simulink model "Main_plasticbike"  (R2022b)
settings: Solver=ode23  StartTime=0.0  StopTime=sim_time-0.02
undefined symbols (not defined in the file): bike_model, bike_params, D_balancing_inner, D_balancing_outer, e1_max, g, I_balancing_inner, I_balancing_outer, initial_state, k1, k2, linearized_sys, P_balancing_inner, P_balancing_outer, pert_deltadot_state, pert_deltadot_state_fun, pert_phidot_state, pert_phidot_state_fun, Psiref, Th, Ts, v, Xref, Yref
libraries: slpidlib x2, cstblocks x1
settings Model: Creator=Hadi Hajieghrary  LastModifiedBy=levi1
settings SolverCC: MaxConsecutiveMinStep=10  ZeroCrossAlgorithm=Adaptive  AlgebraicLoopSolver=TrustRegion  AutoInsertRateTranBlk=on
settings DebuggingCC: AlgebraicLoopMsg=none  UnconnectedInputMsg=warning  UnconnectedOutputMsg=warning  UnconnectedLineMsg=warning
settings ModelReferenceCC: EnableRefExpFcnMdlSchedulingChecks=on
settings RTWCC: DLArmComputeVersion=19.05

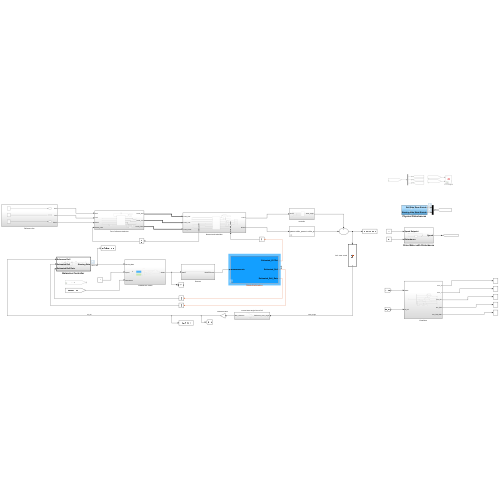
[thumbnail: Simulink's stored preview of the top-level diagram]
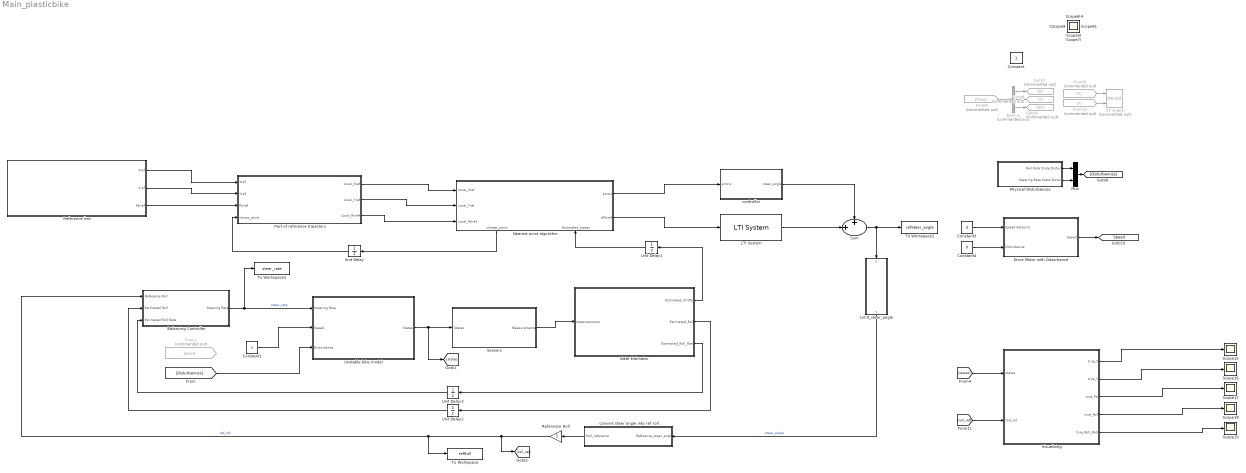
== system Main_plasticbike ==
  "Balancing Controller " : Subsystem  TreatAsAtomicUnit=on  SystemSampleTime=Ts
      settings: MinAlgLoopOccurrences=on
  Constant1 : Constant  Value=v
  Constant3 : Constant  Value=3
  Constant4 : Constant  Value=0
  Demux : Demux  Commented=on  Outputs=3
  Drive Motor with Disturbance : Subsystem
  From1 : From  Commented=on  GotoTag=Speed  TagVisibility=global
  From10 : From  Commented=on  GotoTag=Y
  From8 : From  Commented=on  GotoTag=Pose
  From9 : From  Commented=on  GotoTag=X
  Goto7 : Goto  Commented=on  GotoTag=X
  Goto8 : Goto  Commented=on  GotoTag=Y
  Goto9 : Goto  Commented=on  GotoTag=psi
  LTI System : cstblocks/LTI System  sys=tf(1,[bike_params.a/bike_params.b v/bike_params.b])  IC=[]
  Limit_steer_angle : MATLAB Function  TreatAsAtomicUnit=on
  Mux : Mux  Inputs=2
  Nearest point algorithm : Subsystem
      settings: PortSchema="{\"entries\":[{\"content\":{\"sides\":[{\"content\":{\"connectorIds\":[\"In1\",\"In2\",\"In3\"]},\"type\":\"ConnectorPlacement.EquallySpacedRectSide\",\"uuid\":\"cc846df4-97c1-4e38-a551-63d96742d514\"},{\"content\":{\"connectorIds\":[\"Out1\",\"Out2\"],\"side\":\"RIGHT\"},\"type\":\"ConnectorPlacement.EquallySpacedRectSide\",\"uuid\":\"926eeee4-c51a-40d9-a9a1-df7a0c76cd55\"},{\"content\":{\"connectorIds\":[],\"side\":\"TOP\"},\"type\":\"ConnectorPlacement.EquallySpacedRectSide\",\"uuid\":\"e902e63c-5309-44b2-99e1-76b44c06d1f2\"},{\"content\":{\"connectorIds\":[\"Out3\",\"In4\"],\"side\":\"BOTTOM\"},\"type\":\"ConnectorPlacement.EquallySpacedRectSide\",\"uuid\":\"f92d60b4-b11f-4907-83c4-1907c5b6c496\"}]},\"type\":\"ConnectorPlacement.EquallySpacedConnector\",\"uuid\":\"17b67b4e-0a47-44a6-bf11-0cf8a9b1982c\"}],\"packageUris\":[\"http://schema.mathworks.com/mf0/Connector/R2020b\"],\"version\":\"1.0\"}"
  Part of reference trajectory : Subsystem
  Physical Disturbances : Subsystem
  Reference Roll : Gain
  Reference line : Subsystem
  Scope{,1..19} (20 alike) : Scope
  Sensors : Subsystem
  State Estimator : Subsystem  mask{Parameters=bike_params, Initial_State=initial_state}
      mask prompts: Initial_State "Initial State"
  Sum : Sum  Inputs=++|
  To Workspace : ToWorkspace  VariableName=refRoll  SaveFormat=Timeseries  SampleTime=-1
  To Workspace1 : ToWorkspace  VariableName=refSteer_angle  SaveFormat=Timeseries  SampleTime=-1
  To Workspace2 : ToWorkspace  VariableName=steer_rate  SaveFormat=Timeseries  SampleTime=-1
  Unit Delay : UnitDelay  InitialCondition=1  SampleTime=Ts  HasFrameUpgradeWarning=on
  Unit Delay1 : UnitDelay  InitialCondition=[initial_state.x,initial_state.y,initial_state.heading]  SampleTime=Ts  HasFrameUpgradeWarning=on
  Unit Delay2 : UnitDelay  InitialCondition=initial_state.roll  SampleTime=Ts  HasFrameUpgradeWarning=on
  Unit Delay3 : UnitDelay  InitialCondition=initial_state.roll_rate  SampleTime=Ts  HasFrameUpgradeWarning=on
  Unstable bike model : Subsystem
  Visualizing : Subsystem
  XY Graph : Record  Commented=on  FileSettingsInternal="{\"entries\":[{\"content\":{\"excelSettings\":{\"content\":{},\"type\":\"Streamout.ExcelSettings\"}},\"type\":\"Streamout.FileSettingStorage\",\"uuid\":\"b0b94e94-796c-45bd-bc66-13715b3cee68\"}],\"packageUris\":[\"http://schema.mathworks.com/mf0/streamout_blocks/R2020a\"],\"version\":\"1.0\"}"  Layout=[1 1]  SignalsInternal="{\"entries\":[{\"content\":{\"signals\":[]},\"type\":\"RecordBlkView.InputSignals\",\"uuid\":\"7ae09d58-3f85-47c3-a863-15e07ca78b5f\"}],\"packageUris\":[\"http://schema.mathworks.com/mf0/streamout_blocks/R2020a\"],\"version\":\"1.0\"}"  VisualizationBindings="{\"xyplotplugin\":{\"info\":[{\"series\":[],\"subplotID\":1}]}}"  CompatibilityTag=XY
  controller : Subsystem
  convert steer angle into ref roll : Subsystem
  Constant : Constant  IOType=siggen
  tag scope: Speed=global
  wires:
  From8/1 -> Demux/1
  Demux/1 -> Goto7/1
  Demux/2 -> Goto8/1
  Demux/3 -> Goto9/1
  From10/1 -> XY Graph/2
  From9/1 -> XY Graph/1
  Physical Disturbances/1(Roll Rate State Disturb) -> Mux/1
  Physical Disturbances/2(Steering Rate State Disturb) -> Mux/2
  Mux/1 -> [Disturbances]
  Drive Motor with Disturbance/1(Speed) -> [Speed]
  Constant3/1 -> Drive Motor with Disturbance/1(Speed Setpoint)
  Constant4/1 -> Drive Motor with Disturbance/2(Disturbance)
  "Balancing Controller "/1(Steering Rate) -> Unstable bike model/1(Steering Rate), To Workspace2/1  "steer_rate"
  Reference line/1(Xref) -> Part of reference trajectory/1(Xref)
  Part of reference trajectory/1(Local_Xref) -> Nearest point algorithm/1(Local_Xref)
  Nearest point algorithm/3(closest_point) -> Unit Delay/1
  Nearest point algorithm/1(errors) -> controller/1(errors)
  Unit Delay/1 -> Part of reference trajectory/4(closes_point)
  controller/1(steer_angle) -> Sum/1
  LTI System/1 -> Sum/2
  Nearest point algorithm/2(dPsiref) -> LTI System/1
  Sum/1 -> Limit_steer_angle/1(u), To Workspace1/1
  Limit_steer_angle/1(y) -> convert steer angle into ref roll/1(Reference_steer_angle)  "steer_angle"
  convert steer angle into ref roll/1(Roll_reference) -> Reference Roll/1
  Reference Roll/1 -> [roll_ref], To Workspace/1, "Balancing Controller "/1(Reference Roll)  "ref_roll"
  [Disturbances] -> Unstable bike model/3(Disturbance)
  State Estimator/1(Estimated_X/Y/Psi) -> Unit Delay1/1
  State Estimator/2(Estimated_Roll) -> Unit Delay2/1
  State Estimator/3(Estimated_Roll_Rate) -> Unit Delay3/1
  Sensors/1(Measurements) -> State Estimator/1(measurements)
  Part of reference trajectory/2(Local_Yref) -> Nearest point algorithm/2(Local_Yref)
  Part of reference trajectory/3(Local_Psiref) -> Nearest point algorithm/3(Local_Psiref)
  Reference line/3(Psiref) -> Part of reference trajectory/3(Psiref)
  [states] -> Visualizing/1(states)
  Visualizing/1(true_X) -> Scope15/1
  Visualizing/2(true_Y) -> Scope16/1
  Visualizing/3(true_Psi) -> Scope17/1
  Visualizing/4(true_Roll) -> Scope18/1
  Visualizing/5(true_Roll_Rate) -> Scope19/1
  Unit Delay1/1 -> Nearest point algorithm/4(Estimated_states)
  Unit Delay2/1 -> "Balancing Controller "/2(Estimated Roll)
  Unit Delay3/1 -> "Balancing Controller "/3(Estimated Roll Rate)
  Reference line/2(Yref) -> Part of reference trajectory/2(Yref)
  [roll_ref] -> Visualizing/2(roll_ref)
  Unstable bike model/1(States) -> [states], Sensors/1(States)
  Constant1/1 -> Unstable bike model/2(Speed)

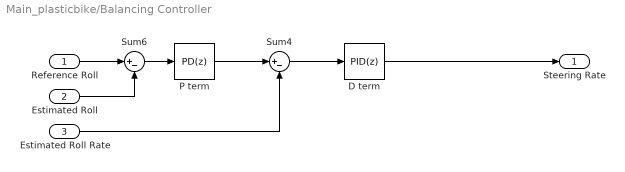
== system Main_plasticbike/Balancing Controller  ==
  Reference Roll : Inport
  Estimated Roll : Inport  Port=2
  Estimated Roll Rate : Inport  Port=3
  D term : slpidlib/PID Controller  Controller=PID  Form=Parallel  TimeDomain=Discrete-time  UseExternalTs=off  SampleTime=Ts  IntegratorMethod=Forward Euler  FilterMethod=Forward Euler  ControllerParametersSource=internal  P=P_balancing_inner  I=I_balancing_inner  UseKiTs=off  D=D_balancing_inner  N=100  UseFilter=off  TunerSelectOption=Transfer Function Based (PID Tuner App)  InitialConditionSource=internal  InitialConditionForIntegrator=0  InitialConditionForFilter=0  DifferentiatorICPrevScaledInput=0  ExternalReset=none  TrackingMode=off  Kt=1  LimitOutput=off  SatLimitsSource=internal  UpperSaturationLimit=inf  LowerSaturationLimit=-inf  LinearizeAsGain=on  AntiWindupMode=none  Kb=1  LimitIntegrator=off  UpperIntegratorSaturationLimit=inf  LowerIntegratorSaturationLimit=-inf  POutMin=[]  POutMax=[]  IOutMin=[]  IOutMax=[]  DOutMin=[]  DOutMax=[]  NOutMin=[]  NOutMax=[]  SumOutMin=[]  SumOutMax=[]  SaturationOutMin=[]  SaturationOutMax=[]  PParamMin=[]  PParamMax=[]  IParamMin=[]  IParamMax=[]  DParamMin=[]  DParamMax=[]  NParamMin=[]  NParamMax=[]  KbParamMin=[]  KbParamMax=[]  KtParamMin=[]  KtParamMax=[]  KbOutMin=[]  KbOutMax=[]  KtOutMin=[]  KtOutMax=[]  IntegratorOutMin=[]  IntegratorOutMax=[]  FilterOutMin=[]  FilterOutMax=[]  SumI1OutMin=[]  SumI1OutMax=[]  SumI2OutMin=[]  SumI2OutMax=[]  SumI3OutMin=[]  SumI3OutMax=[]  SumI4OutMin=[]  SumI4OutMax=[]  SumDOutMin=[]  SumDOutMax=[]  DifferentiatorOutMin=[]  DifferentiatorOutMax=[]  FilterDiffOutCoefMin=[]  FilterDiffOutCoefMax=[]  ReciprocalOutMin=[]  ReciprocalOutMax=[]  SumDenOutMin=[]  SumDenOutMax=[]  SumNumOutMin=[]  SumNumOutMax=[]  DivideOutMin=[]  DivideOutMax=[]  UdiffTsProdOutMin=[]  UdiffTsProdOutMax=[]  NTsProdOutMin=[]  NTsProdOutMax=[]  UintegralTsProdOutMin=[]  UintegralTsProdOutMax=[]  UngainTsProdOutMin=[]  UngainTsProdOutMax=[]  IntegratorContinuousStateAttributes=''  IntegratorStateMustResolveToSignalObject=off  IntegratorRTWStateStorageClass=Auto  FilterContinuousStateAttributes=''  FilterStateMustResolveToSignalObject=off  FilterRTWStateStorageClass=Auto  ParallelPVariant=InternalParameters  IdealPVariant=Disabled  IVariant=InternalParameters  DVariant=InternalParameters  IntegratorVariant=Discrete  SatVariant=Disabled  AWVariant=Passthrough  PCopyVariant=Disabled  TRVariant=Disabled  FdbkBlocksVariant=Forward  IdealPFdbkVariant=Disabled  SatFdbkVariant=Disabled  DerivativeFilterVariant=Differentiator  NVariant=Passthrough  NCopyVariant=Disabled_SignalSpec  FilterICVariant=InternalICsDifferentiator  IntegratorICVariant=InternalICs  ExternalResetVariant=Disabled  TRSumVariant=Passthrough  SumFdbkVariant=Disabled  SumVariant=Sum_PID  TsampFilterVariant=InternalTs  TsampNgainVariant=Passthrough  TsampIntegralVariant=Passthrough  ExternalSaturationOutDataTypeStr=Inherit: Same as second input
  P term : slpidlib/PID Controller  Controller=PD  Form=Parallel  TimeDomain=Discrete-time  UseExternalTs=off  SampleTime=Ts  IntegratorMethod=Forward Euler  FilterMethod=Forward Euler  ControllerParametersSource=internal  P=P_balancing_outer  I=I_balancing_outer  UseKiTs=off  D=D_balancing_outer  N=100  UseFilter=off  TunerSelectOption=Transfer Function Based (PID Tuner App)  InitialConditionSource=internal  InitialConditionForIntegrator=0  InitialConditionForFilter=0  DifferentiatorICPrevScaledInput=0  ExternalReset=none  TrackingMode=off  Kt=1  LimitOutput=off  SatLimitsSource=internal  UpperSaturationLimit=inf  LowerSaturationLimit=-inf  LinearizeAsGain=on  AntiWindupMode=none  Kb=1  LimitIntegrator=off  UpperIntegratorSaturationLimit=inf  LowerIntegratorSaturationLimit=-inf  POutMin=[]  POutMax=[]  IOutMin=[]  IOutMax=[]  DOutMin=[]  DOutMax=[]  NOutMin=[]  NOutMax=[]  SumOutMin=[]  SumOutMax=[]  SaturationOutMin=[]  SaturationOutMax=[]  PParamMin=[]  PParamMax=[]  IParamMin=[]  IParamMax=[]  DParamMin=[]  DParamMax=[]  NParamMin=[]  NParamMax=[]  KbParamMin=[]  KbParamMax=[]  KtParamMin=[]  KtParamMax=[]  KbOutMin=[]  KbOutMax=[]  KtOutMin=[]  KtOutMax=[]  IntegratorOutMin=[]  IntegratorOutMax=[]  FilterOutMin=[]  FilterOutMax=[]  SumI1OutMin=[]  SumI1OutMax=[]  SumI2OutMin=[]  SumI2OutMax=[]  SumI3OutMin=[]  SumI3OutMax=[]  SumI4OutMin=[]  SumI4OutMax=[]  SumDOutMin=[]  SumDOutMax=[]  DifferentiatorOutMin=[]  DifferentiatorOutMax=[]  FilterDiffOutCoefMin=[]  FilterDiffOutCoefMax=[]  ReciprocalOutMin=[]  ReciprocalOutMax=[]  SumDenOutMin=[]  SumDenOutMax=[]  SumNumOutMin=[]  SumNumOutMax=[]  DivideOutMin=[]  DivideOutMax=[]  UdiffTsProdOutMin=[]  UdiffTsProdOutMax=[]  NTsProdOutMin=[]  NTsProdOutMax=[]  UintegralTsProdOutMin=[]  UintegralTsProdOutMax=[]  UngainTsProdOutMin=[]  UngainTsProdOutMax=[]  IntegratorContinuousStateAttributes=''  IntegratorStateMustResolveToSignalObject=off  IntegratorRTWStateStorageClass=Auto  FilterContinuousStateAttributes=''  FilterStateMustResolveToSignalObject=off  FilterRTWStateStorageClass=Auto  ParallelPVariant=InternalParameters  IdealPVariant=Disabled  IVariant=Disabled  DVariant=InternalParameters  IntegratorVariant=Disabled  SatVariant=Disabled  AWVariant=Disabled  PCopyVariant=Disabled  TRVariant=Disabled  FdbkBlocksVariant=Forward  IdealPFdbkVariant=Disabled  SatFdbkVariant=Disabled  DerivativeFilterVariant=Differentiator  NVariant=Passthrough  NCopyVariant=Disabled_SignalSpec  FilterICVariant=InternalICsDifferentiator  IntegratorICVariant=Disabled  ExternalResetVariant=Disabled  TRSumVariant=Passthrough  SumFdbkVariant=Disabled  SumVariant=Sum_PD  TsampFilterVariant=InternalTs  TsampNgainVariant=Passthrough  TsampIntegralVariant=Disabled_SignalSpec  ExternalSaturationOutDataTypeStr=Inherit: Same as second input
  Sum4 : Sum  Inputs=|+-
  Sum6 : Sum  Inputs=|+-
  Steering Rate : Outport
  wires:
  Sum4/1 -> D term/1
  Reference Roll/1 -> Sum6/1
  Sum6/1 -> P term/1
  Estimated Roll Rate/1 -> Sum4/2
  P term/1 -> Sum4/1
  D term/1 -> Steering Rate/1
  Estimated Roll/1 -> Sum6/2

== system Main_plasticbike/Drive Motor with Disturbance ==
  Speed Setpoint : Inport
  Disturbance : Inport  Port=2
  Sum2 : Sum  Inputs=++|
  Transfer Fcn : TransferFcn  Denominator=[2 1]
  Speed : Outport
  wires:
  Sum2/1 -> Speed/1
  Transfer Fcn/1 -> Sum2/2
  Speed Setpoint/1 -> Transfer Fcn/1
  Disturbance/1 -> Sum2/1

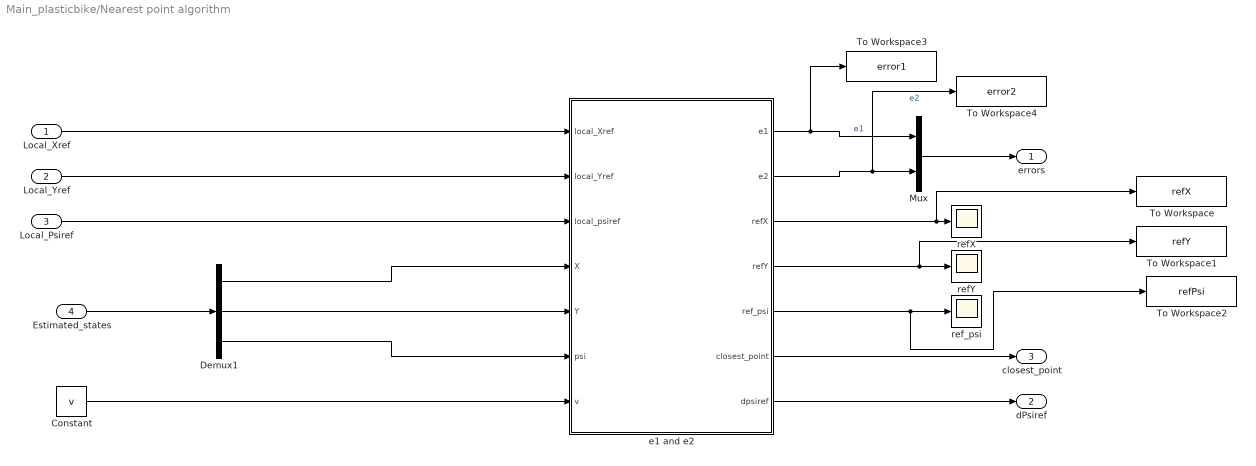
== system Main_plasticbike/Nearest point algorithm ==
  Local_Xref : Inport
  Local_Yref : Inport  Port=2
  Local_Psiref : Inport  Port=3
  Estimated_states : Inport  Port=4
  Constant : Constant  Value=v
  Demux1 : Demux  Outputs=3
  Mux : Mux  Inputs=2
  To Workspace : ToWorkspace  VariableName=refX  SaveFormat=Timeseries  SampleTime=-1
  To Workspace1 : ToWorkspace  VariableName=refY  SaveFormat=Timeseries  SampleTime=-1
  To Workspace2 : ToWorkspace  VariableName=refPsi  SaveFormat=Timeseries  SampleTime=-1
  To Workspace3 : ToWorkspace  VariableName=error1  SaveFormat=Timeseries  SampleTime=-1
  To Workspace4 : ToWorkspace  VariableName=error2  SaveFormat=Timeseries  SampleTime=-1
  e1 and e2 : Subsystem
  refX : Scope
  refY : Scope
  ref_psi : Scope
  errors : Outport
  dPsiref : Outport  Port=2
  closest_point : Outport  Port=3
  wires:
  Estimated_states/1 -> Demux1/1
  Demux1/2 -> e1 and e2/5(Y)
  Demux1/1 -> e1 and e2/4(X)
  Demux1/3 -> e1 and e2/6(psi)
  Constant/1 -> e1 and e2/7(v)
  e1 and e2/1(e1) -> To Workspace3/1, Mux/1  "e1"
  e1 and e2/2(e2) -> To Workspace4/1, Mux/2  "e2"
  Mux/1 -> errors/1
  e1 and e2/6(closest_point) -> closest_point/1
  e1 and e2/3(refX) -> To Workspace/1, refX/1
  e1 and e2/4(refY) -> To Workspace1/1, refY/1
  e1 and e2/5(ref_psi) -> To Workspace2/1, ref_psi/1
  e1 and e2/7(dpsiref) -> dPsiref/1
  Local_Xref/1 -> e1 and e2/1(local_Xref)
  Local_Yref/1 -> e1 and e2/2(local_Yref)
  Local_Psiref/1 -> e1 and e2/3(local_psiref)

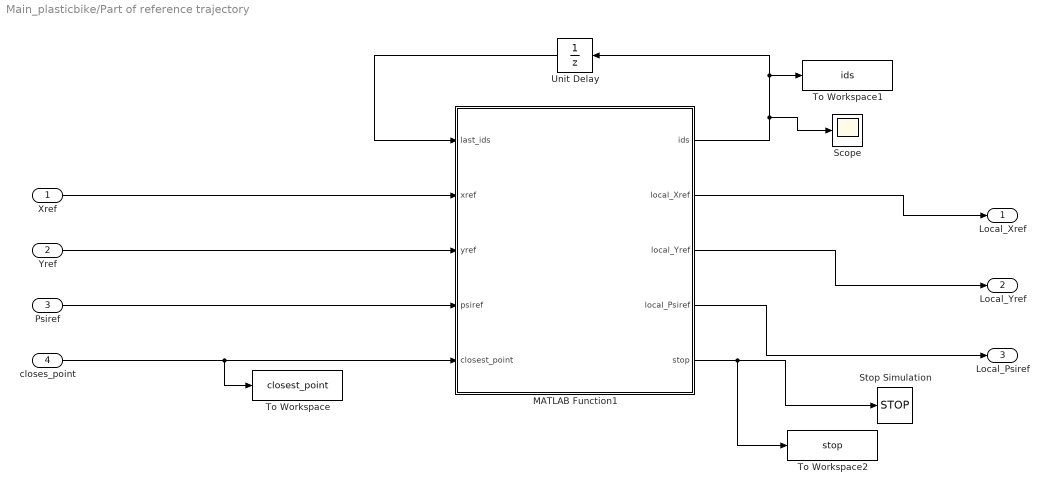
== system Main_plasticbike/Part of reference trajectory ==
  Xref : Inport
  Yref : Inport  Port=2
  Psiref : Inport  Port=3
  closes_point : Inport  Port=4
  MATLAB Function1 : MATLAB Function  TreatAsAtomicUnit=on
  Scope : Scope
  Stop Simulation : Stop
  To Workspace : ToWorkspace  VariableName=closest_point  SaveFormat=Timeseries  SampleTime=-1
  To Workspace1 : ToWorkspace  VariableName=ids  SaveFormat=Timeseries  SampleTime=-1
  To Workspace2 : ToWorkspace  VariableName=stop  SaveFormat=Timeseries  SampleTime=-1
  Unit Delay : UnitDelay  InitialCondition=1  SampleTime=Ts  HasFrameUpgradeWarning=on
  Local_Xref : Outport
  Local_Yref : Outport  Port=2
  Local_Psiref : Outport  Port=3
  wires:
  MATLAB Function1/1(ids) -> Scope/1, To Workspace1/1, Unit Delay/1
  Unit Delay/1 -> MATLAB Function1/1(last_ids)
  closes_point/1 -> To Workspace/1, MATLAB Function1/5(closest_point)
  MATLAB Function1/2(local_Xref) -> Local_Xref/1
  MATLAB Function1/3(local_Yref) -> Local_Yref/1
  MATLAB Function1/4(local_Psiref) -> Local_Psiref/1
  Xref/1 -> MATLAB Function1/2(xref)
  Yref/1 -> MATLAB Function1/3(yref)
  Psiref/1 -> MATLAB Function1/4(psiref)
  MATLAB Function1/5(stop) -> To Workspace2/1, Stop Simulation/1

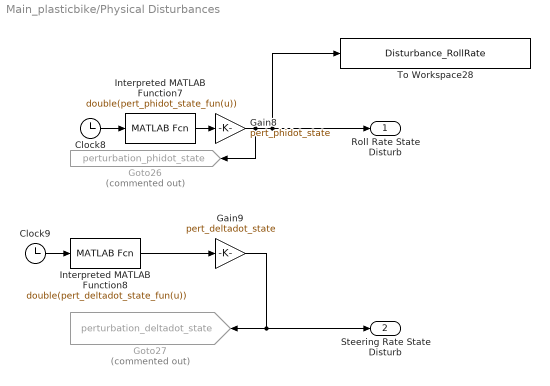
== system Main_plasticbike/Physical Disturbances ==
  Clock8 : Clock
  Clock9 : Clock
  Gain8 : Gain  Gain=pert_phidot_state
  Gain9 : Gain  Gain=pert_deltadot_state
  Goto26 : Goto  Commented=on  GotoTag=perturbation_phidot_state  TagVisibility=global
  Goto27 : Goto  Commented=on  GotoTag=perturbation_deltadot_state  TagVisibility=global
  Interpreted MATLAB Function7 : MATLABFcn  MATLABFcn=double(pert_phidot_state_fun(u))
  Interpreted MATLAB Function8 : MATLABFcn  MATLABFcn=double(pert_deltadot_state_fun(u))
  To Workspace28 : ToWorkspace  VariableName=Disturbance_RollRate  SaveFormat=Timeseries  SampleTime=-1
  Roll Rate State Disturb : Outport
  Steering Rate State Disturb : Outport  Port=2
  wires:
  Interpreted MATLAB Function7/1 -> Gain8/1
  Clock8/1 -> Interpreted MATLAB Function7/1
  Gain8/1 -> Goto26/1, Roll Rate State Disturb/1, To Workspace28/1
  Interpreted MATLAB Function8/1 -> Gain9/1
  Clock9/1 -> Interpreted MATLAB Function8/1
  Gain9/1 -> Steering Rate State Disturb/1, Goto27/1

== system Main_plasticbike/Reference line ==
  Constant : Constant  Value=Xref
  Constant1 : Constant  Value=Yref
  Constant2 : Constant  Value=Psiref
  Xref : Outport
  Yref : Outport  Port=2
  Psiref : Outport  Port=3
  wires:
  Constant/1 -> Xref/1
  Constant1/1 -> Yref/1
  Constant2/1 -> Psiref/1

== system Main_plasticbike/Sensors ==
  States : Inport
  Measurements : Outport
  wires:
  States/1 -> Measurements/1

== system Main_plasticbike/State Estimator ==
  measurements : Inport
  Demux : Demux  Outputs=5
  Mux : Mux  Inputs=3
  Estimated_X/Y/Psi : Outport  VectorParamsAs1DForOutWhenUnconnected=off
  Estimated_Roll : Outport  Port=2  VectorParamsAs1DForOutWhenUnconnected=off
  Estimated_Roll_Rate : Outport  Port=3  VectorParamsAs1DForOutWhenUnconnected=off
  wires:
  Mux/1 -> Estimated_X/Y/Psi/1
  Demux/1 -> Mux/1
  Demux/2 -> Mux/2
  Demux/3 -> Mux/3
  Demux/4 -> Estimated_Roll/1
  Demux/5 -> Estimated_Roll_Rate/1
  measurements/1 -> Demux/1

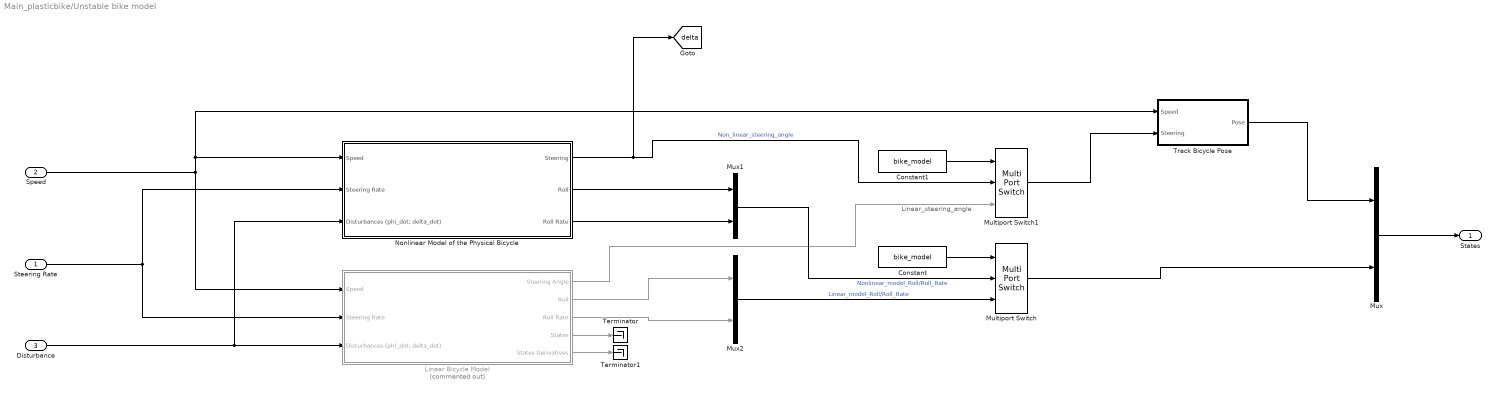
== system Main_plasticbike/Unstable bike model ==
  note: Linear_steering_angle
  Steering Rate : Inport
  Speed : Inport  Port=2
  Disturbance : Inport  Port=3
  Constant : Constant  Value=bike_model
  Constant1 : Constant  Value=bike_model
  Linear Bicycle Model : Subsystem  Commented=on  mask{Parameters=bike_params, linearized_sys=linearized_sys, Initial_State=initial_state}
      mask prompts: linearized_sys "Linearized System"; Initial_State "Initial State"
  Multiport Switch : MultiPortSwitch  Inputs=2  SaturateOnIntegerOverflow=off  InputSameDT=off
  Multiport Switch1 : MultiPortSwitch  Inputs=2  SaturateOnIntegerOverflow=off  InputSameDT=off
  Mux : Mux  Inputs=2
  Mux1 : Mux  Inputs=2
  Mux2 : Mux  Inputs=2
  Nonlinear Model of the Physical Bicycle : Subsystem  mask{Parameters=bike_params, Initial_State=initial_state}
      mask prompts: Initial_State "Initial State"
  Terminator : Terminator
  Terminator1 : Terminator
  "Track Bicycle Pose " : Subsystem  mask{Parameters=bike_params, Initial_State=initial_state}
      mask prompts: Initial_State "Initial State"
  States : Outport
  tag scope: delta=global
  wires:
  Steering Rate/1 -> Linear Bicycle Model/2(Steering Rate), Nonlinear Model of the Physical Bicycle/2(Steering Rate)
  Multiport Switch1/1 -> "Track Bicycle Pose "/2(Steering)
  Constant/1 -> Multiport Switch/1
  Nonlinear Model of the Physical Bicycle/2(Roll) -> Mux1/1
  Nonlinear Model of the Physical Bicycle/3(Roll Rate) -> Mux1/2
  Nonlinear Model of the Physical Bicycle/1(Steering) -> [delta], Multiport Switch1/2  "Non_linear_steering_angle"
  Linear Bicycle Model/2(Roll) -> Mux2/1
  Linear Bicycle Model/3(Roll Rate) -> Mux2/2
  Linear Bicycle Model/1(Steering Angle) -> Multiport Switch1/3
  Mux1/1 -> Multiport Switch/2  "Nonlinear_model_Roll/Roll_Rate"
  Mux2/1 -> Multiport Switch/3  "Linear_model_Roll/Roll_Rate"
  Constant1/1 -> Multiport Switch1/1
  Mux/1 -> States/1
  Multiport Switch/1 -> Mux/2
  "Track Bicycle Pose "/1(Pose) -> Mux/1
  Speed/1 -> Linear Bicycle Model/1(Speed), "Track Bicycle Pose "/1(Speed), Nonlinear Model of the Physical Bicycle/1(Speed)
  Disturbance/1 -> Nonlinear Model of the Physical Bicycle/3(Disturbances (phi_dot; delta_dot)), Linear Bicycle Model/3(Disturbances (phi_dot; delta_dot))
  Linear Bicycle Model/4(States) -> Terminator/1
  Linear Bicycle Model/5(States Derivatives) -> Terminator1/1

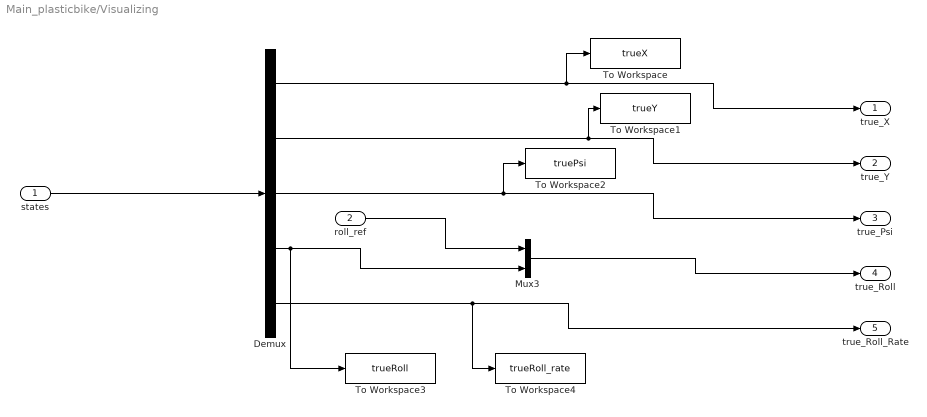
== system Main_plasticbike/Visualizing ==
  states : Inport
  roll_ref : Inport  Port=2
  Demux : Demux  Outputs=5
  Mux3 : Mux  Inputs=2
  To Workspace : ToWorkspace  VariableName=trueX  SaveFormat=Timeseries  SampleTime=-1
  To Workspace1 : ToWorkspace  VariableName=trueY  SaveFormat=Timeseries  SampleTime=-1
  To Workspace2 : ToWorkspace  VariableName=truePsi  SaveFormat=Timeseries  SampleTime=-1
  To Workspace3 : ToWorkspace  VariableName=trueRoll  SaveFormat=Timeseries  SampleTime=-1
  To Workspace4 : ToWorkspace  VariableName=trueRoll_rate  SaveFormat=Timeseries  SampleTime=-1
  true_X : Outport
  true_Y : Outport  Port=2
  true_Psi : Outport  Port=3
  true_Roll : Outport  Port=4
  true_Roll_Rate : Outport  Port=5
  wires:
  states/1 -> Demux/1
  Demux/1 -> true_X/1, To Workspace/1
  Demux/3 -> To Workspace2/1, true_Psi/1
  roll_ref/1 -> Mux3/1
  Demux/4 -> To Workspace3/1, Mux3/2
  Mux3/1 -> true_Roll/1
  Demux/5 -> To Workspace4/1, true_Roll_Rate/1
  Demux/2 -> To Workspace1/1, true_Y/1

== system Main_plasticbike/controller ==
  errors : Inport
  Constant : Constant  Value=k1
  Constant1 : Constant  Value=k2
  Constant2 : Constant  Value=e1_max
  Demux : Demux  Outputs=2
  MATLAB Function4 : MATLAB Function  TreatAsAtomicUnit=on
  steer_angle : Outport
  wires:
  errors/1 -> Demux/1
  Demux/1 -> MATLAB Function4/3(e1)
  Demux/2 -> MATLAB Function4/4(e2)
  Constant1/1 -> MATLAB Function4/2(k2)
  Constant/1 -> MATLAB Function4/1(k1)
  Constant2/1 -> MATLAB Function4/5(e1_max)
  MATLAB Function4/1(steer_angle) -> steer_angle/1

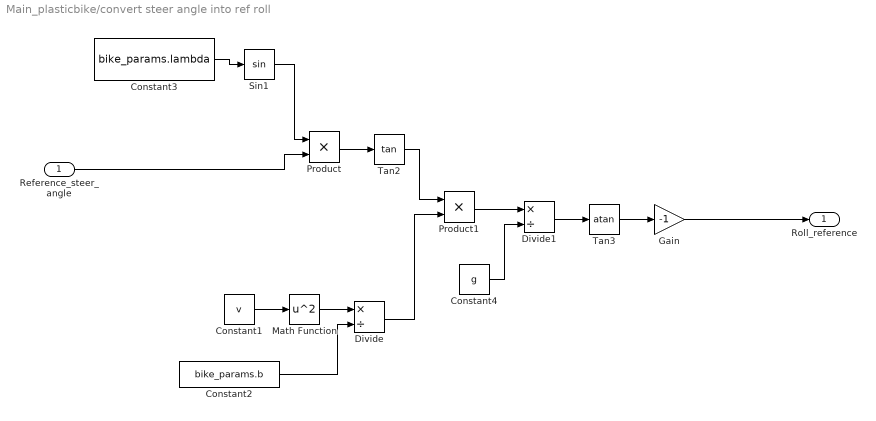
== system Main_plasticbike/convert steer angle into ref roll ==
  Reference_steer_angle : Inport
  Constant1 : Constant  Value=v  SampleTime=Ts
  Constant2 : Constant  Value=bike_params.b  SampleTime=Ts
  Constant3 : Constant  Value=bike_params.lambda  SampleTime=Ts
  Constant4 : Constant  Value=g  SampleTime=Ts
  Divide : Product  Inputs=*/
  Divide1 : Product  Inputs=*/
  Gain : Gain  Gain=-1
  Math Function : Math  Operator=square
  Product : Product
  Product1 : Product
  Sin1 : Trigonometry
  Tan2 : Trigonometry  Operator=tan
  Tan3 : Trigonometry  Operator=atan
  Roll_reference : Outport
  wires:
  Product/1 -> Tan2/1
  Constant2/1 -> Divide/2
  Reference_steer_angle/1 -> Product/2
  Product1/1 -> Divide1/1
  Constant1/1 -> Math Function/1
  Constant3/1 -> Sin1/1
  Constant4/1 -> Divide1/2
  Divide/1 -> Product1/2
  Math Function/1 -> Divide/1
  Divide1/1 -> Tan3/1
  Gain/1 -> Roll_reference/1
  Sin1/1 -> Product/1
  Tan2/1 -> Product1/1
  Tan3/1 -> Gain/1

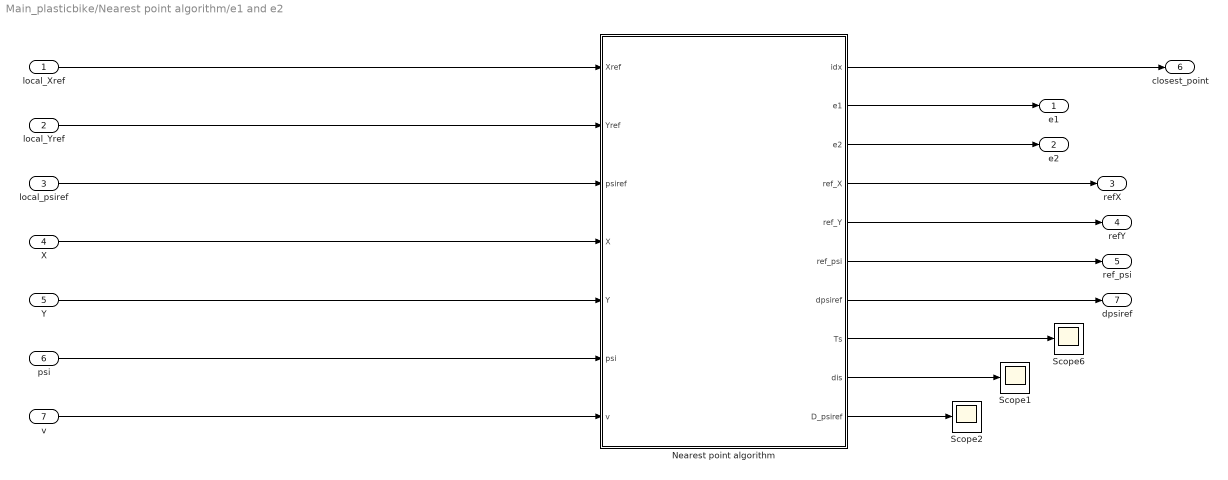
== system Main_plasticbike/Nearest point algorithm/e1 and e2 ==
  local_Xref : Inport
  local_Yref : Inport  Port=2
  local_psiref : Inport  Port=3
  X : Inport  Port=4
  Y : Inport  Port=5
  psi : Inport  Port=6
  v : Inport  Port=7
  Nearest point algorithm : MATLAB Function  TreatAsAtomicUnit=on
  Scope1 : Scope
  Scope2 : Scope
  Scope6 : Scope
  e1 : Outport
  e2 : Outport  Port=2
  refX : Outport  Port=3
  refY : Outport  Port=4
  ref_psi : Outport  Port=5
  closest_point : Outport  Port=6
  dpsiref : Outport  Port=7
  wires:
  Nearest point algorithm/6(ref_psi) -> ref_psi/1
  Nearest point algorithm/5(ref_Y) -> refY/1
  Nearest point algorithm/4(ref_X) -> refX/1
  psi/1 -> Nearest point algorithm/6(psi)
  Y/1 -> Nearest point algorithm/5(Y)
  Nearest point algorithm/3(e2) -> e2/1
  Nearest point algorithm/2(e1) -> e1/1
  X/1 -> Nearest point algorithm/4(X)
  local_Yref/1 -> Nearest point algorithm/2(Yref)
  local_psiref/1 -> Nearest point algorithm/3(psiref)
  local_Xref/1 -> Nearest point algorithm/1(Xref)
  Nearest point algorithm/1(idx) -> closest_point/1
  v/1 -> Nearest point algorithm/7(v)
  Nearest point algorithm/7(dpsiref) -> dpsiref/1
  Nearest point algorithm/8(Ts) -> Scope6/1
  Nearest point algorithm/9(dis) -> Scope1/1
  Nearest point algorithm/10(D_psiref) -> Scope2/1

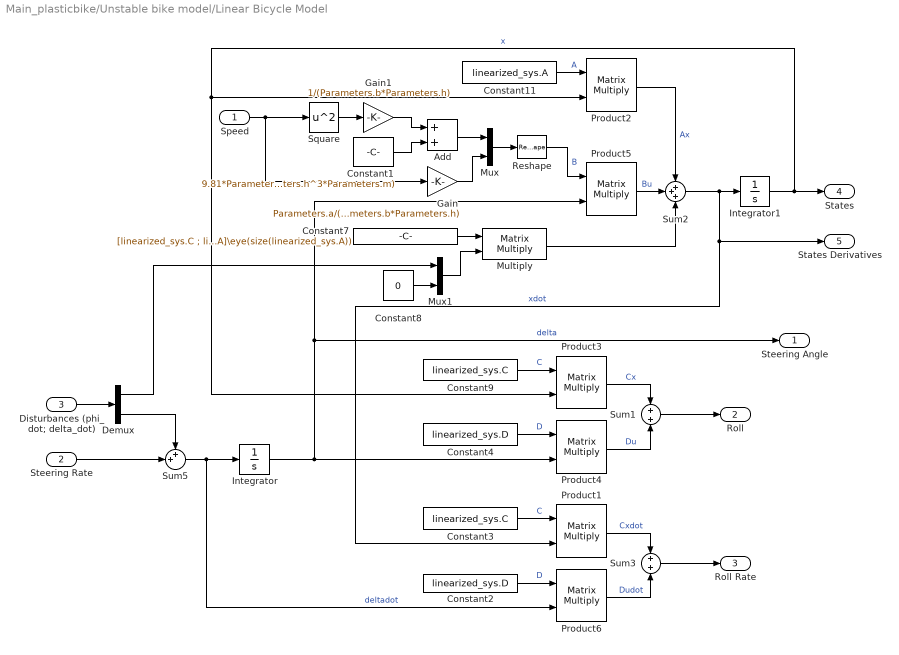
== system Main_plasticbike/Unstable bike model/Linear Bicycle Model ==
  Speed : Inport
  Steering Rate : Inport  Port=2
  Disturbances (phi_dot; delta_dot) : Inport  Port=3
  Add : Sum
  Constant1 : Constant  Value=9.81*Parameters.inertia_front/(Parameters.h^3*Parameters.m)
  Constant11 : Constant  Value=linearized_sys.A  VectorParams1D=off
  Constant2 : Constant  Value=linearized_sys.D  VectorParams1D=off
  Constant3 : Constant  Value=linearized_sys.C  VectorParams1D=off
  Constant4 : Constant  Value=linearized_sys.D  VectorParams1D=off
  Constant7 : Constant  Value=[linearized_sys.C ; linearized_sys.C*linearized_sys.A]\eye(size(linearized_sys.A))  VectorParams1D=off
  Constant8 : Constant  Value=0
  Constant9 : Constant  Value=linearized_sys.C  VectorParams1D=off
  Demux : Demux  Outputs=2
  Gain : Gain  Gain=Parameters.a/(Parameters.b*Parameters.h)
  Gain1 : Gain  Gain=1/(Parameters.b*Parameters.h)
  Integrator : Integrator  InitialCondition=Initial_State.steering
  Integrator1 : Integrator  InitialCondition=[linearized_sys.C ; linearized_sys.C*linearized_sys.A]\[Initial_State.roll ; Initial_State.roll_rate]
  Multiply : Product  Multiplication=Matrix(*)
  Mux : Mux  Inputs=2
  Mux1 : Mux  Inputs=2
  Product{1..6} (6 alike) : Product  SCDEnableBlockLinearizationSpecification=on  Multiplication=Matrix(*)
  Reshape : Reshape  OutputDimensionality=Customize  OutputDimensions=[size(linearized_sys.B,1),size(linearized_sys.B,2)]
  Square : Math  Operator=square  SignedPower=on
  Sum1 : Sum
  Sum2 : Sum  Inputs=+++
  Sum3 : Sum
  Sum5 : Sum  Inputs=++|
  Steering Angle : Outport  VectorParamsAs1DForOutWhenUnconnected=off
  Roll : Outport  Port=2  VectorParamsAs1DForOutWhenUnconnected=off
  Roll Rate : Outport  Port=3  VectorParamsAs1DForOutWhenUnconnected=off
  States : Outport  Port=4  VectorParamsAs1DForOutWhenUnconnected=off
  States Derivatives : Outport  Port=5  VectorParamsAs1DForOutWhenUnconnected=off
  wires:
  Product5/1 -> Sum2/2  "Bu"
  Constant11/1 -> Product2/1  "A"
  Sum2/1 -> Product1/2, States Derivatives/1, Integrator1/1  "xdot"
  Product2/1 -> Sum2/1  "Ax"
  Sum1/1 -> Roll/1
  Reshape/1 -> Product5/1  "B"
  Steering Rate/1 -> Sum5/2
  Product4/1 -> Sum1/2  "Du"
  Product3/1 -> Sum1/1  "Cx"
  Gain1/1 -> Add/1
  Constant1/1 -> Add/2
  Mux/1 -> Reshape/1
  Add/1 -> Mux/1
  Gain/1 -> Mux/2
  Speed/1 -> Square/1, Gain/1
  Square/1 -> Gain1/1
  Disturbances (phi_dot; delta_dot)/1 -> Demux/1
  Sum5/1 -> Integrator/1, Product6/2  "deltadot"
  Multiply/1 -> Sum2/3
  Demux/1 -> Mux1/1
  Constant7/1 -> Multiply/1
  Mux1/1 -> Multiply/2
  Constant8/1 -> Mux1/2
  Demux/2 -> Sum5/1
  Constant9/1 -> Product3/1  "C"
  Constant4/1 -> Product4/1  "D"
  Sum3/1 -> Roll Rate/1
  Integrator1/1 -> States/1, Product2/2, Product3/2  "x"
  Product6/1 -> Sum3/2  "Dudot"
  Constant3/1 -> Product1/1  "C"
  Product1/1 -> Sum3/1  "Cxdot"
  Constant2/1 -> Product6/1  "D"
  Integrator/1 -> Product5/2, Steering Angle/1, Product4/2  "delta"

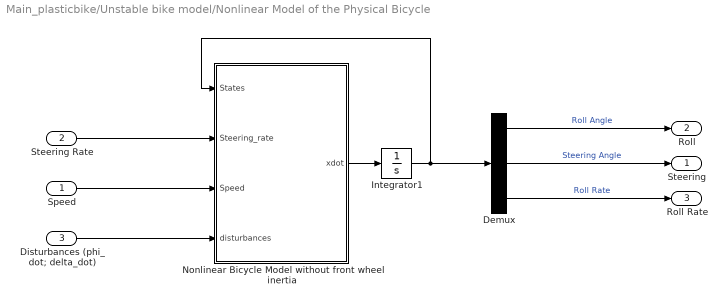
== system Main_plasticbike/Unstable bike model/Nonlinear Model of the Physical Bicycle ==
  Speed : Inport
  Steering Rate : Inport  Port=2
  Disturbances (phi_dot; delta_dot) : Inport  Port=3
  Demux : Demux  Outputs=3
  Integrator1 : Integrator  InitialCondition=[Initial_State.roll ; Initial_State.steering ; Initial_State.roll_rate]
  Nonlinear Bicycle Model without front wheel inertia : MATLAB Function  TreatAsAtomicUnit=on  mask{Parameters=Parameters}
  Steering : Outport  VectorParamsAs1DForOutWhenUnconnected=off
  Roll : Outport  Port=2  VectorParamsAs1DForOutWhenUnconnected=off
  Roll Rate : Outport  Port=3  VectorParamsAs1DForOutWhenUnconnected=off
  wires:
  Integrator1/1 -> Nonlinear Bicycle Model without front wheel inertia/1(States), Demux/1
  Demux/1 -> Roll/1  "Roll Angle"
  Nonlinear Bicycle Model without front wheel inertia/1(xdot) -> Integrator1/1
  Speed/1 -> Nonlinear Bicycle Model without front wheel inertia/3(Speed)
  Demux/3 -> Roll Rate/1  "Roll Rate"
  Demux/2 -> Steering/1  "Steering Angle"
  Steering Rate/1 -> Nonlinear Bicycle Model without front wheel inertia/2(Steering_rate)
  Disturbances (phi_dot; delta_dot)/1 -> Nonlinear Bicycle Model without front wheel inertia/4(disturbances)

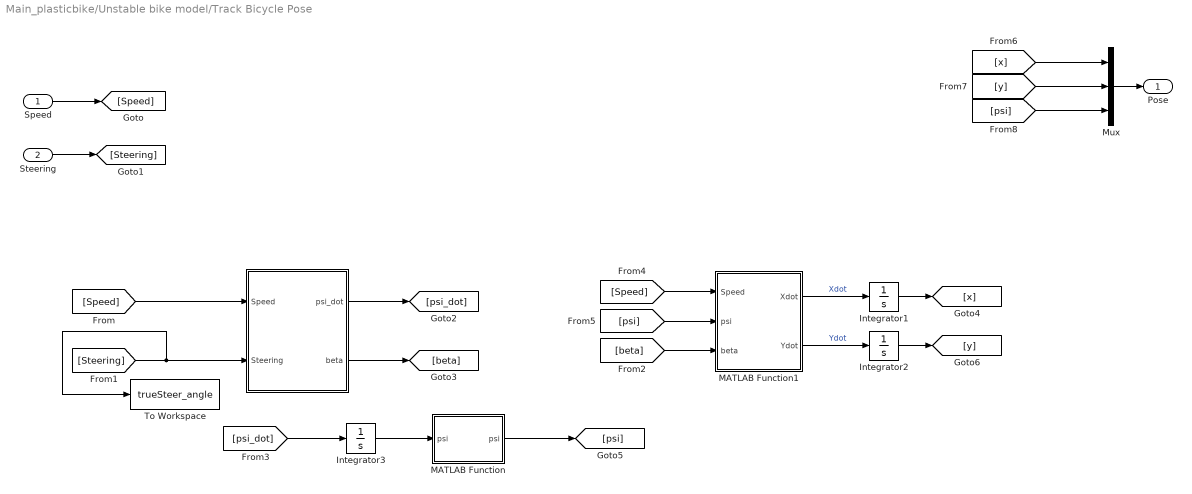
== system Main_plasticbike/Unstable bike model/Track Bicycle Pose  ==
  Speed : Inport
  Steering : Inport  Port=2
  " " : MATLAB Function  TreatAsAtomicUnit=on  mask{Parameters=Parameters}
  Integrator1 : Integrator  InitialCondition=Initial_State.x
  Integrator2 : Integrator  InitialCondition=Initial_State.y
  Integrator3 : Integrator  InitialCondition=Initial_State.heading
  MATLAB Function : MATLAB Function  TreatAsAtomicUnit=on
  MATLAB Function1 : MATLAB Function  TreatAsAtomicUnit=on
  Mux : Mux  Inputs=3
  To Workspace : ToWorkspace  VariableName=trueSteer_angle  SaveFormat=Timeseries  SampleTime=-1
  Pose : Outport
  wires:
  Speed/1 -> [Speed]
  Steering/1 -> [Steering]
  " "/2(beta) -> [beta]
  MATLAB Function1/2(Ydot) -> Integrator2/1  "Ydot"
  MATLAB Function1/1(Xdot) -> Integrator1/1  "Xdot"
  [psi] -> MATLAB Function1/2(psi)
  [psi_dot] -> Integrator3/1
  [Speed] -> MATLAB Function1/1(Speed)
  Integrator3/1 -> MATLAB Function/1("psi ")
  Mux/1 -> Pose/1
  Integrator1/1 -> [x]
  Integrator2/1 -> [y]
  [beta] -> MATLAB Function1/3(beta)
  [x] -> Mux/1
  [y] -> Mux/2
  [psi] -> Mux/3
  " "/1(psi_dot) -> [psi_dot]
  [Steering] -> To Workspace/1, " "/2(Steering)
  [Speed] -> " "/1(Speed)
  MATLAB Function/1(psi) -> [psi]

== matlab function Main_plasticbike/Part of reference trajectory/MATLAB Function1 ==
  data: last_ids input; ids output; xref input; local_Xref output size=Nn [..30000]; local_Yref output size=Nn [..30000]; local_Psiref output size=Nn [..30000]; yref input; psiref input; closest_point input; Ts parameter; Th parameter; v parameter; stop output
function [ids,local_Xref,local_Yref,local_Psiref,stop] = fcn(last_ids,xref,yref,psiref,closest_point, Ts, Th, v)

ids=last_ids+closest_point-1;% calculate the initial index of the points that will be sent to next block

Ns=ceil(Th/Ts);% Th,Ts is definited in "StudentProject2021.m", Ns is the number of points sent to next block
M=ids+Ns;% calculate the end index of the end index that will be sent to next block
n=size(xref,1); % size of whole trajectory points 
if M>n % if reached near end of reference, local trajectry becomes shorter
    M=n;
end
stop = 0;
if ids>=n-(n/50)
    stop = 1;
end
% if ids>=n-1
%     ids=n-2;
% end
bike_dis=v*Ts;
tra_dis=0;
for i=ids:1:M-1 % send the points from index ids:M-1 to next block
    tra_dis=sqrt((xref(i+1,1)-xref(i,1))^2+(yref(i+1,1)-yref(i,1))^2)+tra_dis;
end
if bike_dis>tra_dis %if bike_dis is larger a lot than tra_dis, it's difficult to track reference trajectory, display warning
%     disp('warning');
end


local_Xref=xref(ids:M,1);
local_Yref=yref(ids:M,1);
local_Psiref=psiref(ids:M,1);

== matlab function Main_plasticbike/Limit_steer_angle ==
  data: u input; y output
function y = fcn(u)
% limit steer angle between -pi/4 and pi/4

if u>=pi/4
    u=pi/4;
 
end
if u<=-pi/4
    u=-pi/4;
   
end
y = u;

== matlab function Main_plasticbike/Unstable bike model/Track Bicycle Pose /MATLAB Function ==
  data: psi input; psi output
function psi = fcn(psi)

%psi limit
if psi >= pi
    psi = mod(psi,-2*pi);
end

if psi <= -pi
    psi = mod(psi,2*pi);
end

== matlab function Main_plasticbike/controller/MATLAB Function4 ==
  data: k1 input; k2 input; e1 input; e2 input; steer_angle output; e1_max input
function steer_angle = fcn(k1,k2,e1,e2,e1_max)

delta=-k1*sign(e1)*min(abs(e1),e1_max)-k2*e2;

% delta=-k1*e1-k2*e2;



steer_angle = delta;

== matlab function Main_plasticbike/Unstable bike model/Track Bicycle Pose /MATLAB Function1 ==
  data: Speed input; psi input; Xdot output; beta input; Ydot output
function [Xdot, Ydot]  = fcn(Speed, psi, beta)

Xdot = Speed * cos(psi + beta);
Ydot = Speed * sin(psi + beta);

== matlab function Main_plasticbike/Unstable bike model/Track Bicycle Pose /  ==
  data: Speed input; Steering input; psi_dot output; Parameters parameter; beta output
function [psi_dot, beta] = fcn(Speed, Steering, Parameters)

eff_steering = sin(Parameters.lambda) * Steering;

beta = atan( Parameters.a /Parameters.b * tan(eff_steering) );
psi_dot = (Speed / Parameters.a) * sin(beta);

== matlab function Main_plasticbike/Unstable bike model/Nonlinear Model of the Physical Bicycle/Nonlinear Bicycle Model without front wheel inertia ==
  data: States input; Steering_rate input; Speed input; disturbances input; xdot output; Parameters parameter
function xdot = fcn(States, Steering_rate, Speed, disturbances, Parameters)

g = 9.81;

d_phidot = disturbances(1);
d_deltadot = disturbances(2);

phi = States(1);
delta = States(2);
phi_d = States(3);

% xdot = [phidot deltadot phiddot]
xdot1 = phi_d + d_phidot;
xdot2 = Steering_rate + d_deltadot;
xdot3 = (g/Parameters.h)*sin(phi) + ((Parameters.a*Speed)/(Parameters.b*Parameters.h))/(cos(sin(Parameters.lambda)*delta)^2)*sin(Parameters.lambda)*Steering_rate ...
                                  + ((Parameters.h*Speed^2-g*Parameters.a*Parameters.c)/(Parameters.b*Parameters.h^2))*sin(Parameters.lambda)*tan(delta);

xdot = [xdot1 xdot2 xdot3]';

== matlab function Main_plasticbike/Nearest point algorithm/e1 and e2/Nearest point algorithm ==
  settings: updateMethod=DISCRETE  sampleTime=Ts
  data: idx output; Xref input; e1 output; Yref input; psiref input; X input; Y input; psi input; e2 output; ref_X output; ref_Y output; ref_psi output; dpsiref output; v input; Ts output; dis output; D_psiref output
function [idx,e1,e2,ref_X,ref_Y,ref_psi,dpsiref,Ts,dis,D_psiref]= fcn(Xref,Yref,psiref,X,Y,psi,v)
%% calculations on a local part of the trajectory

n=size(Xref,1);%Xref,Yref,psiref are all "Nx1" vectors, n=N

% % find index of closest point on the trajectory to the bike
% dist=zeros(n,1);
% for i=1:1:n
%     dist(i,1)=sqrt((Xref(i,1)-X)^2+(Yref(i,1)-Y)^2);
% end
% 
% [~,idx]=min(dist); % index of closest point

% Finding the closest point going forward. Stop searching once next
% distance increases
i=1;
while sqrt((Xref(i,1)-X)^2+(Yref(i,1)-Y)^2) >= sqrt((Xref(i+1,1)-X)^2+(Yref(i+1,1)-Y)^2)
i = i+1;
end
idx = i;    % index of closest point

% calculate e1 and e2        
dx = X - Xref(idx,1);
dy = Y - Yref(idx,1);
e1= dy*cos(psiref(idx,1)) - dx*sin(psiref(idx,1));% this make e1 include "direction" automatically
e2=psi-psiref(idx,1);%calculate e2

% closest point on the local trajectory
ref_X=Xref(idx,1);
ref_Y=Yref(idx,1);
ref_psi=psiref(idx,1);

 % keep heading error should be between -pi 2 pi
   e2=mod(e2+pi,2*pi)-pi; 


next_idx=idx+1;% choose idx+1 to calculate dpsiref
if next_idx>=n
    next_idx=n;
end
    
D_psiref=psiref(next_idx,1)-psiref(idx,1);
% To limit D_psiref  between -2pi and 2pi
if D_psiref>=pi
    D_psiref=mod(D_psiref,-2*pi);
end
if D_psiref<=-pi
    D_psiref=mod(D_psiref,2*pi);
end

%calculate the time between psiref(idx,1) and psiref(idx+1,1)
dX=Xref(next_idx,1)-ref_X;
dY=Yref(next_idx,1)-ref_Y;
dis=sqrt(dX^2+dY^2);
Ts=dis/v;

dpsiref=(D_psiref)/Ts;


end
